simulink model "tanque_simulink_disc"  (R2019b)
settings: Solver=VariableStepAuto  StartTime=0.0  StopTime=1000.0  RelTol=1e-3
values from neighbouring files (symbols this model uses):
  A = A /pi^2 /( (rad_menor + h0/tan(ang))^4)    [tanque_simulink_param.m]
  A_tustin = Hld_tustin.A    [tanque_simulink_param.m]
  A_zoh = Hld_zoh.A    [tanque_simulink_param.m]
  ang = pi/3    (= 1.0471975512)    [tanque_simulink_param.m]
  B = (-sqrt(2*g*h0)*(r_apertura^2)) /( (rad_menor + h0/tan(ang))^2)    [tanque_simulink_param.m]
  B_tustin = Hld_tustin.B    [tanque_simulink_param.m]
  B_zoh = Hld_zoh.B    [tanque_simulink_param.m]
  C = 1    [tanque_simulink_param.m]
  C_tustin = Hld_tustin.C    [tanque_simulink_param.m]
  C_zoh = Hld_zoh.C    [tanque_simulink_param.m]
  D = 0    [tanque_simulink_param.m]
  d_p_apertura = 0.05    [tanque_simulink_param.m]
  D_tustin = Hld_tustin.D    [tanque_simulink_param.m]
  D_zoh = Hld_zoh.D    [tanque_simulink_param.m]
  g = 9.8    [tanque_simulink_param.m]
  h0 = 0.6    [tanque_simulink_param.m]
  p_apertura_lin = Q_ent/(pi*r_apertura^2) / (sqrt(2*g*h0))    [tanque_simulink_param.m]
  Q_ent = 0.0035    [tanque_simulink_param.m]
  r_apertura = 0.0254    [tanque_simulink_param.m]
  rad_menor = 0.05    [tanque_simulink_param.m]
  Ts = 10    [tanque_simulink_param.m]
settings Model: Creator=Franco  LastModifiedBy=Franco

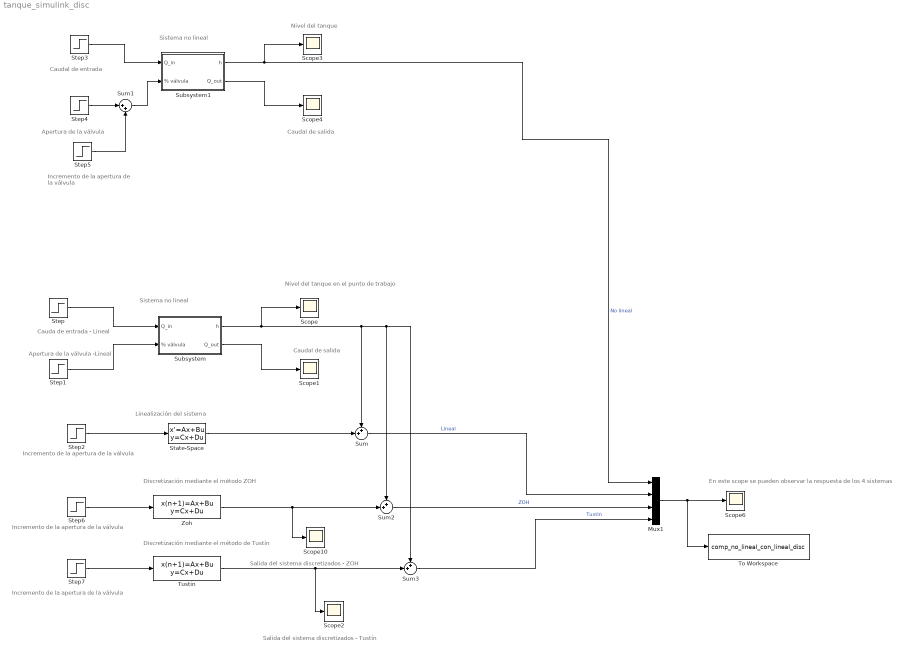
== system tanque_simulink_disc ==
  note: Salida del sistema discretizados - Tustín
  note: Salida del sistema discretizados - ZOH
  note: Incremento de la apertura de la válvula
  note: Incremento de la apertura de la válvula
  note: Incremento de la apertura de la válvula
  note: Caudal de salida
  note: Nivel del tanque en el punto de trabajo
  note: Apertura de la válvula -Lineal
  note: Cauda de entrada - Lineal
  note: Nivel del tanque
  note: Caudal de salida
  note: Incremento de la
      | apertura de la válvula
  note: Apertura de la válvula
  note: Caudal de entrada
  note: Sistema no lineal
  note: Sistema no lineal
  note: Linealización del sistema
  note: En este scope se pueden observar la respuesta de los 4 sistemas
  note: Discretización mediante el método de Tustín
  note: Discretización mediante el método ZOH
  Mux1 : Mux
  Scope{,1..4,6,10} (7 alike) : Scope
  State-Space : StateSpace  A=A  B=B  C=C  D=D  InitialCondition=0
  Step : Step  After=Q_ent  SampleTime=0
  Step1 : Step  After=p_apertura_lin  SampleTime=0
  Step2 : Step  Time=10  After=p_apertura_lin *d_p_apertura  SampleTime=0
  Step3 : Step  After=Q_ent  SampleTime=0
  Step4 : Step  After=p_apertura_lin  SampleTime=0
  Step5 : Step  Time=10  After=p_apertura_lin*d_p_apertura  SampleTime=0
  Step6 : Step  Time=10  After=p_apertura_lin *d_p_apertura  SampleTime=0
  Step7 : Step  Time=10  After=p_apertura_lin *d_p_apertura  SampleTime=0
  Subsystem : Subsystem
  Subsystem1 : Subsystem
  Sum : Sum  Inputs=++|
  Sum1 : Sum  Inputs=|++
  Sum2 : Sum  Inputs=++|
  Sum3 : Sum  Inputs=++|
  To Workspace : ToWorkspace  VariableName=comp_no_lineal_con_lineal_disc  SaveFormat=Timeseries  SampleTime=-1
  Tustin : DiscreteStateSpace  A=A_tustin  B=B_tustin  C=C_tustin  D=D_tustin  SampleTime=Ts
  Zoh : DiscreteStateSpace  A=A_zoh  B=B_zoh  C=C_zoh  D=D_zoh  SampleTime=Ts
  wires:
  Subsystem/1(h) -> Sum3/1, Sum2/1, Sum/1, Scope/1
  Subsystem/2(Q_out) -> Scope1/1
  Step2/1 -> State-Space/1
  State-Space/1 -> Sum/2
  Step3/1 -> Subsystem1/1(Q_in)
  Subsystem1/2(Q_out) -> Scope4/1
  Subsystem1/1(h) -> Mux1/1, Scope3/1  "No lineal"
  Step5/1 -> Sum1/2
  Step4/1 -> Sum1/1
  Sum1/1 -> Subsystem1/2(" % válvula")
  Step1/1 -> Subsystem/2(" % válvula")
  Step/1 -> Subsystem/1(Q_in)
  Step6/1 -> Zoh/1
  Step7/1 -> Tustin/1
  Sum3/1 -> Mux1/4  "Tustin"
  Sum2/1 -> Mux1/3  "ZOH"
  Sum/1 -> Mux1/2  "Lineal"
  Tustin/1 -> Scope2/1, Sum3/2
  Zoh/1 -> Scope10/1, Sum2/2
  Mux1/1 -> To Workspace/1, Scope6/1

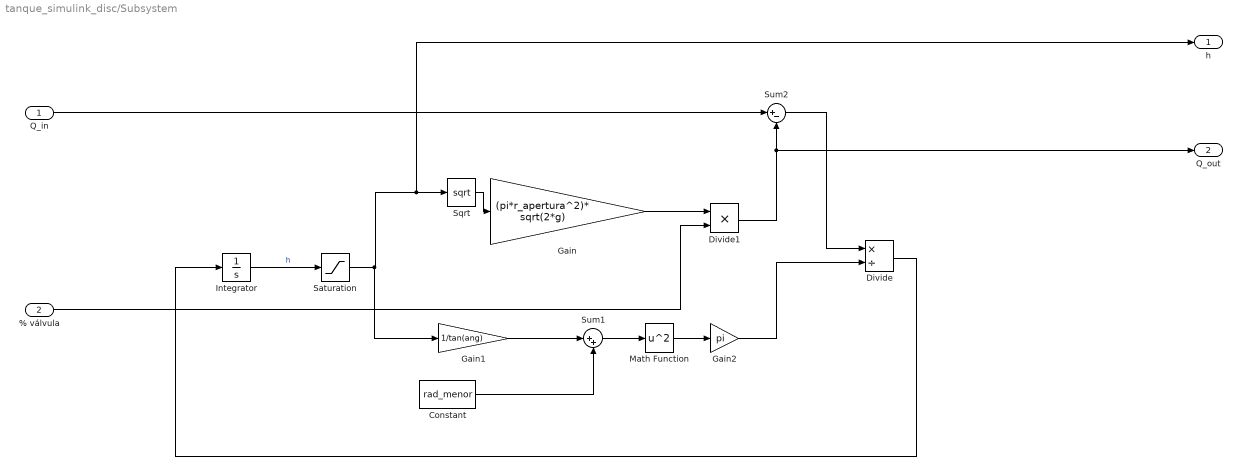
== system tanque_simulink_disc/Subsystem ==
  Q_in : Inport
  " % válvula" : Inport  Port=2
  Constant : Constant  Value=rad_menor
  Divide : Product  Inputs=*/
  Divide1 : Product  Inputs=**
  Gain : Gain  Gain=(pi*r_apertura^2)* sqrt(2*g)
  Gain1 : Gain  Gain=1/tan(ang)
  Gain2 : Gain  Gain=pi
  Integrator : Integrator  InitialCondition=h0
  Math Function : Math  Operator=square  SignedPower=off  SaturateOnIntegerOverflow=on
  Saturation : Saturate  UpperLimit=1  LowerLimit=0
  Sqrt : Sqrt  SaturateOnIntegerOverflow=on
  Sum1 : Sum  Inputs=|++
  Sum2 : Sum  Inputs=|+-
  h : Outport
  Q_out : Outport  Port=2
  wires:
  Gain/1 -> Divide1/1
  Integrator/1 -> Saturation/1  "h"
  Sqrt/1 -> Gain/1
  Sum2/1 -> Divide/1
  Math Function/1 -> Gain2/1
  Saturation/1 -> Gain1/1, h/1, Sqrt/1
  Gain1/1 -> Sum1/1
  Sum1/1 -> Math Function/1
  Divide/1 -> Integrator/1
  Gain2/1 -> Divide/2
  Q_in/1 -> Sum2/1
  Constant/1 -> Sum1/2
  " % válvula"/1 -> Divide1/2
  Divide1/1 -> Q_out/1, Sum2/2

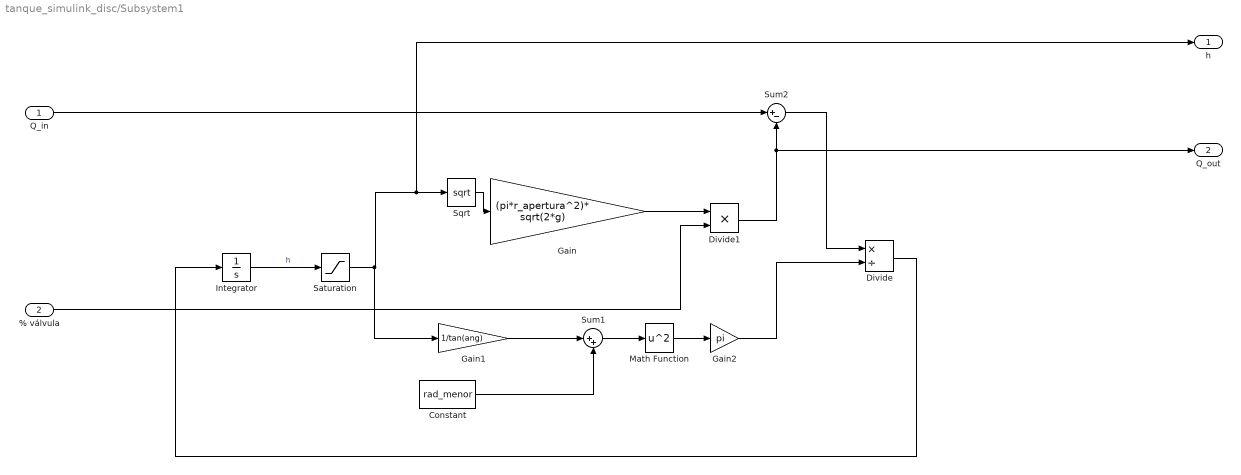
== system tanque_simulink_disc/Subsystem1 ==
  Q_in : Inport
  " % válvula" : Inport  Port=2
  Constant : Constant  Value=rad_menor
  Divide : Product  Inputs=*/
  Divide1 : Product  Inputs=**
  Gain : Gain  Gain=(pi*r_apertura^2)* sqrt(2*g)
  Gain1 : Gain  Gain=1/tan(ang)
  Gain2 : Gain  Gain=pi
  Integrator : Integrator  InitialCondition=h0
  Math Function : Math  Operator=square  SignedPower=off  SaturateOnIntegerOverflow=on
  Saturation : Saturate  UpperLimit=1  LowerLimit=0
  Sqrt : Sqrt  SaturateOnIntegerOverflow=on
  Sum1 : Sum  Inputs=|++
  Sum2 : Sum  Inputs=|+-
  h : Outport
  Q_out : Outport  Port=2
  wires:
  Gain/1 -> Divide1/1
  Integrator/1 -> Saturation/1  "h"
  Sqrt/1 -> Gain/1
  Sum2/1 -> Divide/1
  Math Function/1 -> Gain2/1
  Saturation/1 -> Gain1/1, h/1, Sqrt/1
  Gain1/1 -> Sum1/1
  Sum1/1 -> Math Function/1
  Divide/1 -> Integrator/1
  Gain2/1 -> Divide/2
  Q_in/1 -> Sum2/1
  Constant/1 -> Sum1/2
  " % válvula"/1 -> Divide1/2
  Divide1/1 -> Q_out/1, Sum2/2
